simulink model "AlgoritmoGen"  (R2015a)
settings: Solver=ode45  StartTime=0.0  StopTime=10.0  RelTol=1e-3
values from neighbouring files (symbols this model uses):
  T1 = 0.2    [mainPID.m]
libraries: cstblocks x2
settings Model: Creator=Asus  LastModifiedBy=Asus

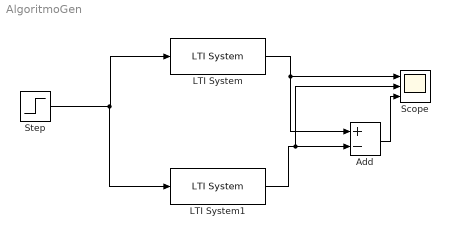
== system AlgoritmoGen ==
  Add : Sum  Inputs=+-
  LTI System : cstblocks/LTI System  sys=tf(1,[T1 1])  IC=[]
  LTI System1 : cstblocks/LTI System  sys=Y  IC=[]
  Scope : Scope  NumInputPorts=3
      settings: YMin=-5~-5~-5  YMax=5~5~5
  Step : Step  SampleTime=0
  wires:
  Step/1 -> LTI System1/1, LTI System/1
  Add/1 -> Scope/3
  LTI System/1 -> Scope/1, Add/1
  LTI System1/1 -> Add/2, Scope/2
